simulink model "px4demo_EKF"  (R2017b)
settings: Solver=ode3  StartTime=0.0  StopTime=inf  FixedStep=Ts  RelTol=1e-3  EnableMultiTasking=on
PostLoadFcn:
  | Ts = 1/250;
InitFcn:
  | alignTime = floor(398.001 * Ts);
  | EAS2TAS = 1;
  | LatDegInit = 1;
  | LngDegInit = 1;
  | msecVelDelay = 300;
  | msecPosDelay = 300;
  | msecHgtDelay = 420;
  | msecMagDelay = 30;
  | msecTasDelay = 200;
undefined symbols (not defined in the file): RGBLED_COLOR_ENUM, RGBLED_MODE_ENUM
libraries: simulink x9, pixhawk_slib_sensors_actuators x3, simulink_need_slupdate x2
(part 4 of 4)

== matlab function px4demo_EKF/EKF/EKF/FuseData/Fuse Vel Pos Measurements ==
  data: states input; P input; accNavMag input; FuseVelData input; VelNED input; StatesAtVelTime input; FusePosData input; PosNE input; StatesAtPosTime input; FuseHgtData input; HgtMea input; nextStates output; nextP output; innovation output; varInnov output; StatesAtHgtTime input; useAirspeed input
%#codegen
function [...
    nextStates, ... % state vector after fusion of measurements (q0, ... , q3, VelN,E,D, PosN,E,D, WindN,E, P0, camera roll pitch yaw misalignment)
    nextP, ... % state covariance matrix after fusion of corrections
    innovation,... % NED velocity and NED position innovations (m/s, m)
    varInnov] ... % NED velocity and NED position innovation variance ((m/s)^2, m^2)
    = FuseVelPosNED( ...
    states, ... % predicted states from the INS (q0, ... , q3, VelN,E,D, PosN,E,D, WindN,E, P0, camera roll pitch yaw misalignment)
    P, ... % predicted covariance
    accNavMag, ... % magnitude of rate of change of velocity in navigation frame (m/s^2)
    FuseVelData, ... % Boolean to initiate fusion of velocity measurements
    VelNED, ... % NED velocity measurements (m/s)
    StatesAtVelTime, ... % States captured at GPs measurement time
    FusePosData,  ... % Boolean to initiate fusion of position measurements
    PosNE, ... % NE position measurements (m)
    StatesAtPosTime, ... % States captured at GPs measurement time
    FuseHgtData, ... % Boolean to initiate fusion of height measurements
    HgtMea, ... % D position measurement (m)
    StatesAtHgtTime, ... % States captured at height measurement time
    useAirspeed) % Boolean to indicate that an airspeed sensor is being used

% define persistent variables
persistent velFailCount;
if isempty(velFailCount)
    velFailCount = uint32(0);
end
persistent posFailCount;
if isempty(posFailCount)
    posFailCount = uint32(0);
end
persistent hgtFailCount;
if isempty(hgtFailCount)
    hgtFailCount = uint32(0);
end

% initialise measurement health flags to false
velHealth = 0;
posHealth = 0;
hgtHealth = 0;

% Specify GPS velocity induced error
velErr = single(0.15*accNavMag);
posErr = single(0.15*accNavMag);
% Specify the GPS and height measurement variances.
R_OBS = single([(0.1^2 + velErr^2) (0.1^2 + velErr^2) (0.1^2 + velErr^2) (2.0^2 + posErr^2) (2.0^2 + posErr^2) 2.0^2]);

% Specify the count before forcing use of GPS or height data after invalid
% data. We need to force GPS again sooner without
% airspeed data as the nav velocities will be unconstrained.
gpsRetryTime = single(30);
gpsRetryTimeNoTAS = single(5);
hgtRetryTime = single(30);
dt = single(0.02);
if useAirspeed
    maxVelFailCount = round(gpsRetryTime/dt);
    maxPosFailCount = maxVelFailCount;
else
    maxVelFailCount = round(gpsRetryTimeNoTAS/dt);
    maxPosFailCount = maxVelFailCount;
end
maxHgtFailCount = round(hgtRetryTime/dt);

% initialise the innovation vector
innovation = single(zeros(6,1));

% initialise the innovation variance vector
varInnov = single(zeros(6,1));

% Define the observation vector
observation = single([VelNED;PosNE;-HgtMea]);

% Perform sequential fusion of GPS and height measurements. This assumes that the
% errors in the dfferent velocity and position componenets are
% uncorrelated which is not true, however in the absence of covariance
% data from the GPS receiver it is the only assumption we can make
% so we might as well take advantage of the computational efficiencies
% associated with sequential fusion
if (FuseVelData || FusePosData || FuseHgtData)
    % calculate innovation variances
    for obsIndex = 1:6
        stateIndex = 4 + obsIndex;
        varInnov(obsIndex) = P(stateIndex,stateIndex) + R_OBS(obsIndex);
    end
    % calculate innovations and check validity against limits
    if FuseVelData
        velInnov = StatesAtVelTime(5:7) - VelNED;
        if (velInnov(1)*velInnov(1) + velInnov(2)*velInnov(2) + velInnov(3)*velInnov(3)) < 25.0*(varInnov(1) + varInnov(2) + varInnov(3)) || ...
                (velFailCount > maxVelFailCount)
            velHealth = 1;
            velFailCount = uint32(0);
        else
            velHealth = 0;
            velFailCount = velFailCount + uint32(1);
        end
    end
    if FusePosData
        posInnov = StatesAtPosTime(8:9) - PosNE;
        if (posInnov(1)*posInnov(1) + posInnov(2)*posInnov(2)) < 100.0*(varInnov(4) + varInnov(5)) || ...
                (posFailCount > maxPosFailCount)
            posHealth = 1;
            posFailCount = uint32(0);
        else
            posHealth = 0;
            posFailCount = posFailCount + uint32(1);
        end
    end
    if FusePosData
        hgtInnov = StatesAtHgtTime(10) + HgtMea;
        if (hgtInnov*hgtInnov) < 25.0*varInnov(6) || ...
                (hgtFailCount > maxHgtFailCount)
            hgtHealth = 1;
            hgtFailCount = uint32(0);
        else
            hgtHealth = 0;
            hgtFailCount = hgtFailCount + uint32(1);
        end
    end
    % Set range for sequential fusion of velocity and position measurements
    fuseData = zeros(1,6);
    if FuseVelData
        fuseData(1) = 1;
        fuseData(2) = 1;
        fuseData(3) = 1;
    end
    if FusePosData
        fuseData(4) = 1;
        fuseData(5) = 1;
    end
    if FuseHgtData
        fuseData(6) = 1;
    end
    % Fuse measurements sequentially
    for obsIndex = 1:6
        if fuseData(obsIndex)
            % Apply data health checks
            % If no airspeed data, start using GPS data after x seconds
            if (velHealth && (obsIndex >= 1 && obsIndex <= 3)) || ...
                    (posHealth && (obsIndex == 4 || obsIndex == 5)) || ...
                    (hgtHealth && (obsIndex == 6))
                stateIndex = 4 + obsIndex;
                % Calculate the measurement innovation, using states from the
                % appropriate time coordinate
                if (obsIndex >= 1 && obsIndex <= 3)
                    innovation(obsIndex) = StatesAtVelTime(stateIndex) - observation(obsIndex);
                elseif (obsIndex == 4 || obsIndex == 5)
                    innovation(obsIndex) = StatesAtPosTime(stateIndex) - observation(obsIndex);
                elseif (obsIndex == 6)
                    innovation(obsIndex) = StatesAtHgtTime(stateIndex) - observation(obsIndex);
                else
                    innovation(obsIndex) = 0.0;
                end
                
                % Calculate the Kalman Gain
                varInnov(obsIndex) = P(stateIndex,stateIndex) + R_OBS(obsIndex); % data logging only
                SK = 1/varInnov(obsIndex);
                K = P(:,stateIndex)*SK;
                % Calculate state corrections
                xk = K * innovation(obsIndex);
                % Update the covariance - take advantage of direct observation of a
                % single state at stateIndex
                %P = (I - K*H)*P;
                KHP = single(zeros(24,24));
                for rowIndex = 1:24
                    for colIndex = 1:24
                        KHP(rowIndex,colIndex) = K(rowIndex)*P(stateIndex,colIndex);
                    end
                end
                P = P - KHP;
                % Apply the state corrections and re-normaliase the quaternions
                states = states - xk;
                % Normalise the quaternion states
                quatMag = sqrt(states(1)^2 + states(2)^2 + states(3)^2 + states(4)^2);
                if (quatMag > 1e-12)
                    states(1:4) = states(1:4) / quatMag;
                end
            end
        end
    end
end
% Output covariance matrix and state vector
nextP = P;
nextStates = states;
end
